simulink subsystem "Motor"  (R2023a)
settings: Solver=VariableStepAuto  StartTime=0.0  StopTime=10.0  RelTol=1e-3
undefined symbols (not defined in the file or in its folder): b, J, K, L, R
settings Model: Creator=MY PC  LastModifiedBy=MY PC

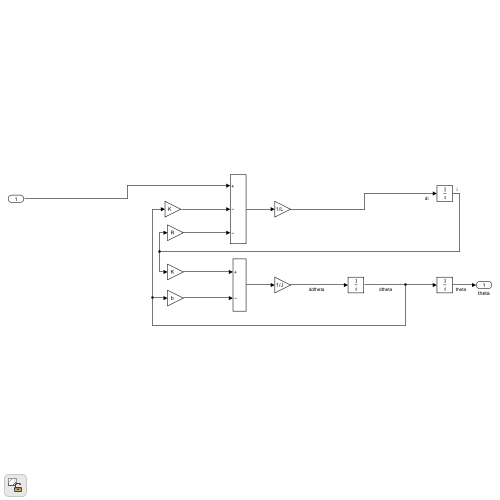
[thumbnail: Simulink's stored preview of the top-level diagram]
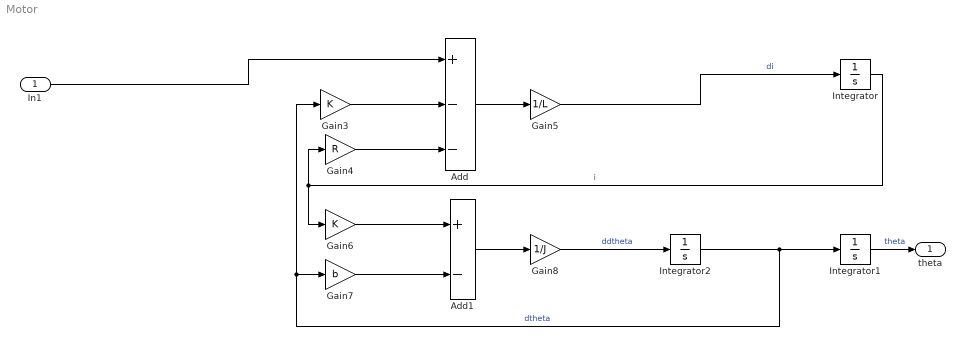
== system Motor ==
  In1 : Inport
  Add : Sum  Inputs=+--
  Add1 : Sum  Inputs=+-
  Gain3 : Gain  Gain=K
  Gain4 : Gain  Gain=R
  Gain5 : Gain  Gain=1/L
  Gain6 : Gain  Gain=K
  Gain7 : Gain  Gain=b
  Gain8 : Gain  Gain=1/J
  Integrator : Integrator
  Integrator1 : Integrator
  Integrator2 : Integrator
  theta : Outport
  wires:
  Add/1 -> Gain5/1
  Integrator2/1 -> Integrator1/1, Gain3/1, Gain7/1  "dtheta"
  Gain8/1 -> Integrator2/1  "ddtheta"
  Integrator/1 -> Gain6/1, Gain4/1  "i"
  Gain3/1 -> Add/2
  Gain6/1 -> Add1/1
  Gain4/1 -> Add/3
  Gain7/1 -> Add1/2
  Gain5/1 -> Integrator/1  "di"
  Add1/1 -> Gain8/1
  Integrator1/1 -> theta/1  "theta"
  In1/1 -> Add/1
